simulink model "ModelC"  (R2018a)
settings: Solver=ode23  StartTime=0.0  StopTime=0.25  MaxStep=10e-6  RelTol=1e-3
libraries: powerlib x16
settings Model: Creator=ivank  LastModifiedBy=ivank
settings SolverCC: InitialStep=10e-8

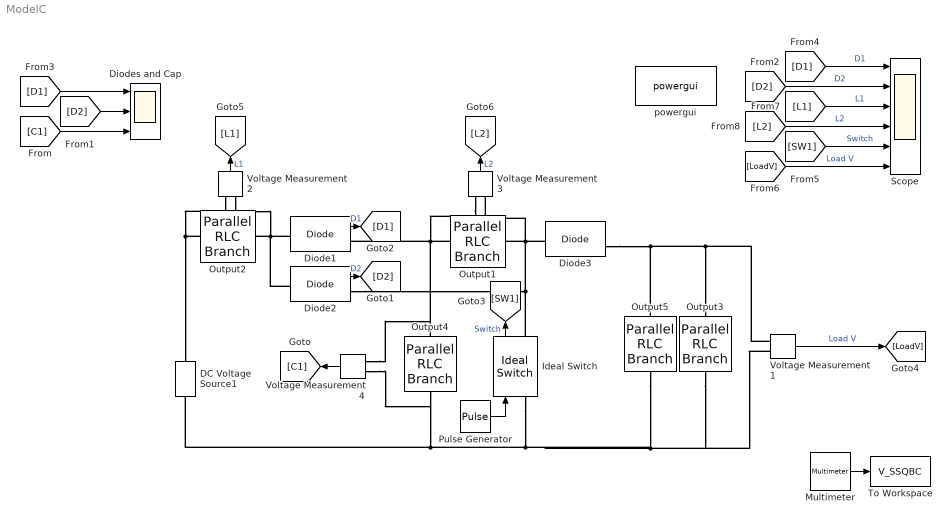
== system ModelC ==
  DC Voltage Source1 : powerlib/Electrical Sources/DC Voltage Source  Amplitude=10  Measurements=None
  Diode1 : powerlib/Power Electronics/Diode  Ron=0.001  Lon=0  Vf=0.  IC=0  UseSnubber=0  Rs=500  Cs=250e-9  Measurements=on
  Diode2 : powerlib/Power Electronics/Diode  Ron=0.001  Lon=0  Vf=0  IC=0  UseSnubber=0  Rs=500  Cs=250e-9  Measurements=on
  Diode3 : powerlib/Power Electronics/Diode  Ron=0.001  Lon=0  Vf=0.  IC=0  UseSnubber=0  Rs=500  Cs=250e-9  Measurements=on
  Diodes and Cap : Scope  NumInputPorts=3
  Ideal Switch : powerlib/Power Electronics/Ideal Switch  Ron=0.001  Lon=0  IC=0  Rs=1e5  Cs=inf  Measurements=on
  Multimeter : powerlib/Measurements/Multimeter  PhasorSimulation=off  OutputType=Complex  sel=3  L=10  Gain=1  yselected={'Ub: Output3'};  PSBOutputType=1  PSBequivalent=0  AxesSetting=[0,0.1,-100,100]  Display=0  SavedBlockNames=-11
  Output1 : powerlib/Elements/Parallel RLC Branch  LConnTagsString=a  RConnTagsString=__new0  BranchType=L  Resistance=7.225  Inductance=150e-6  SetiL0=off  InitialCurrent=0  Capacitance=100*10e-6  Setx0=off  InitialVoltage=0  Measurements=Branch voltage and current
  Output2 : powerlib/Elements/Parallel RLC Branch  LConnTagsString=a  RConnTagsString=__new0  BranchType=L  Resistance=7.225  Inductance=150e-6  SetiL0=off  InitialCurrent=0  Capacitance=100*10e-6  Setx0=off  InitialVoltage=0  Measurements=Branch voltage and current
  Output3 : powerlib/Elements/Parallel RLC Branch  LConnTagsString=a  RConnTagsString=__new0  BranchType=R  Resistance=125  Inductance=1e-3  SetiL0=off  InitialCurrent=0  Capacitance=100*10e-6  Setx0=off  InitialVoltage=0  Measurements=Branch voltage and current
  Output4 : powerlib/Elements/Parallel RLC Branch  LConnTagsString=a  RConnTagsString=__new0  BranchType=C  Resistance=7.225  Inductance=1e-3  SetiL0=off  InitialCurrent=0  Capacitance=220e-6  Setx0=off  InitialVoltage=0  Measurements=Branch voltage and current
  Output5 : powerlib/Elements/Parallel RLC Branch  LConnTagsString=a  RConnTagsString=__new0  BranchType=C  Resistance=7.225  Inductance=1e-3  SetiL0=off  InitialCurrent=0  Capacitance=220e-6  Setx0=off  InitialVoltage=0  Measurements=Branch voltage and current
  Pulse Generator : DiscretePulseGenerator  PulseType=Time based  Period=1/50000  PulseWidth=60
  Scope : Scope  NumInputPorts=6
  To Workspace : ToWorkspace  VariableName=V_SSQBC  SaveFormat=Timeseries  SampleTime=-1
  Voltage Measurement{1..4} (4 alike) : powerlib/Measurements/Voltage Measurement  PhasorSimulation=off  OutputType=Complex  PSBequivalent=0
  powergui : powerlib/powergui  Priority=1  SimulationMode=Continuous  SampleTime=50e-6  frequency=60  Iterations=50  frequencyindice=0  Pbase=100e6  ErrMax=1e-4  UnitsV=kV  UnitsW=MW  buscounter=0  FunctionMessages=off  echomessages=off  EnableUseOfTLC=off  CurrentSourceSwitches=off  DisableSnubberDevices=off  DisableRonSwitches=off  DisableVfSwitches=off  DisplayEquations=off  SolverType=Tustin/Backward Euler (TBE)  Interpol=off  ExternalGateDelay=off  methode=off  Ts=100  x0status=blocks  SPID=on  SwTol=0  HookPort=off  RestoreLinks=warning  ResistiveCurrentMeasurement=off  Frange=[0:2:500]  Ylog=off  Xlog=on  ShowGrid=off  save=off  variable=ZData  structure=0  ZoomFFT=off  StartTime=0.0  cycles=1  DisplayStyle=1  fundamental=60  FreqAxis=off  MaxFrequency=1000  frequencyindicesteady=1  RmsSteady=1  display=off
  wires:
  [LoadV] -> Scope/6  "Load V"
  Pulse Generator/1 -> Ideal Switch/1
  [L1] -> Scope/3  "L1"
  [L2] -> Scope/4  "L2"
  [SW1] -> Scope/5  "Switch"
  Voltage Measurement4/1 -> [C1]
  [C1] -> Diodes and Cap/3
  Diode2/1 -> [D2]  "D2"
  [D2] -> Diodes and Cap/2
  [D2] -> Scope/2  "D2"
  Diode1/1 -> [D1]  "D1"
  [D1] -> Diodes and Cap/1
  [D1] -> Scope/1  "D1"
  Ideal Switch/1 -> [SW1]  "Switch"
  Voltage Measurement1/1 -> [LoadV]  "Load V"
  Voltage Measurement2/1 -> [L1]  "L1"
  Voltage Measurement3/1 -> [L2]  "L2"
  Multimeter/1 -> To Workspace/1
  connections:
  Ideal Switch/LConn1 -- Output5/RConn1 -- Output3/RConn1 -- Voltage Measurement1/LConn2 -- Voltage Measurement4/LConn2 -- Output4/RConn1 -- DC Voltage Source1/LConn1
  Output2/RConn1 -- Voltage Measurement2/LConn2 -- DC Voltage Source1/RConn1
  Diode1/LConn1 -- Diode2/LConn1 -- Voltage Measurement2/LConn1 -- Output2/LConn1
  Output1/RConn1 -- Voltage Measurement4/LConn1 -- Output4/LConn1 -- Diode1/RConn1 -- Voltage Measurement3/LConn2
  Ideal Switch/RConn1 -- Diode2/RConn1 -- Diode3/LConn1 -- Voltage Measurement3/LConn1 -- Output1/LConn1
  Voltage Measurement1/LConn1 -- Output3/LConn1 -- Output5/LConn1 -- Diode3/RConn1
